simulink model "problem1"  (R2020a)
settings: Solver=VariableStepAuto  StartTime=0.0  StopTime=10.0  RelTol=1e-3
settings Model: Creator=kasutav  LastModifiedBy=kasutav

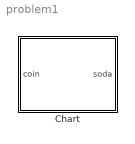
== system problem1 ==
  Chart : Stateflow chart  TreatAsAtomicUnit=on

== stateflow chart problem1/Chart ==
  state coin_check
  state coin_5
  state coin_10
  (default) -> coin_check
  coin_check -> coin_5 : [coin==1]{soda=0}
  coin_5 -> coin_check [order 1] : [coin==2]{soda=1}
  coin_10 -> coin_check [order 2]
  coin_10 -> coin_5 [order 1] : [coin==2]{soda=1}
  coin_5 -> coin_10 [order 2] : [coin==1]{soda=0}
  data: coin input; soda output
